simulink model "soccer_strategy"  (R2018a)
settings: Solver=FixedStepDiscrete  StartTime=0.0  StopTime=inf  FixedStep=0.01  RelTol=1e-3
InitFcn:
  | soccer_strategy_setup
model workspace (MAT data in the model file):
  SL_ROS_VariableLengthArrays_MaxSizes.CommonInfo.ArrayTruncateAction = 'EmitWarning'
  SL_ROS_VariableLengthArrays_MaxSizes.MsgTypeMap = containers.Map
  SL_ROS_VariableLengthArrays_MaxSizes.MsgTypeMap.serialization.keys = {'sensor_msgs/Image'}
  SL_ROS_VariableLengthArrays_MaxSizes.MsgTypeMap.serialization.values{1}(1).PropertyName = 'Data'
  SL_ROS_VariableLengthArrays_MaxSizes.MsgTypeMap.serialization.values{1}(1).DataType = 'uint8'
  SL_ROS_VariableLengthArrays_MaxSizes.MsgTypeMap.serialization.values{1}(1).MaxLength = 921600
  SL_ROS_VariableLengthArrays_MaxSizes.MsgTypeMap.serialization.values{1}(2).PropertyName = 'Encoding'
  SL_ROS_VariableLengthArrays_MaxSizes.MsgTypeMap.serialization.values{1}(2).DataType = 'uint8'
  SL_ROS_VariableLengthArrays_MaxSizes.MsgTypeMap.serialization.values{1}(2).MaxLength = 128
  SL_ROS_VariableLengthArrays_MaxSizes.MsgTypeMap.serialization.uniformity = 0
  SL_ROS_VariableLengthArrays_MaxSizes.MsgTypeMap.serialization.keyType = 'char'
  SL_ROS_VariableLengthArrays_MaxSizes.MsgTypeMap.serialization.valueType = 'any'
  ctrlParam1 = 1
  ctrlParam2 = 1.5
  sampleTime = 0.01
values from neighbouring files (symbols this model uses):
  feetGain = 0.1    [soccer_strategy_setup.m]
  forearmGain = 1.5    [soccer_strategy_setup.m]
  hipCalveGain = 1    [soccer_strategy_setup.m]
  kneeGain = 2    [soccer_strategy_setup.m]
  motorCalibration = [      0;      0;      0.05;     0.05;      0;      0;      0;      0;      0;      0;      0;      0;      0;      0;      0;      0;      0;      0;      0;      0]    [soccer_strategy_calibration.m]    (also in soccer_strategy_setup.m = [0;0;0;0;0;0;0;0;0;0;0;0;0;0;0;0;0;0;0;0])
undefined symbols (not defined in the file or in its folder): DiscIntNeverNeededParam, manual, ready, ready_armsback, standing
libraries: robotlib x8, dspsrcs4 x7, simulink x4, simulink_extras x3, robotcorelib x1
settings Model: Creator=scastro  LastModifiedBy=daniel
settings OptimizationCC: PassReuseOutputArgsAs=Individual arguments  EfficientMapNaN2IntZero=off  MaxStackSize=64
settings DebuggingCC: ParameterTunabilityLossMsg=error
settings HardwareCC: ProdBitPerPointer=32  ProdBitPerSizeT=32  ProdBitPerPtrDiffT=32  ProdLargestAtomicFloat=None  ProdIntDivRoundTo=Undefined  ProdEndianess=Unspecified  ProdWordSize=32  ProdHWDeviceType=Generic->Unspecified (assume 32-bit Generic)  TargetBitPerLong=64  TargetBitPerPointer=64  TargetBitPerSizeT=64  TargetBitPerPtrDiffT=64  TargetLongLongMode=on  TargetIntDivRoundTo=Zero  TargetEndianess=LittleEndian  TargetWordSize=64  TargetHWDeviceType=MATLAB Host  ProdEqTarget=off
settings RTWCC: SystemTargetFile=ert.tlc  HardwareBoard=Robot Operating System (ROS)  TLCOptions="-aInlineSetEventsForThisBaseRateFcn=TLC_FALSE -aSuppressMultiTaskScheduler=TLC_FALSE  -aRateBasedStepFcn=0"  TemplateMakefile=ert_default_tmf  GenerateReport=on  Toolchain=Catkin  IncludeHyperlinkInReport=on  LaunchReport=on  TargetLang=C++  GenerateTraceInfo=on  GenerateTraceReport=on  GenerateTraceReportSl=on  GenerateTraceReportSf=on  GenerateTraceReportEml=on
settings CodeAppCC: ForceParamTrailComments=on  IgnoreCustomStorageClasses=off  MaxIdLength=128  OperatorAnnotations=on  SimulinkDataObjDesc=on  SFDataObjDesc=on  InsertBlockDesc=on
settings ERTTargetCC: MultiInstanceERTCode=on  CodeInterfacePackaging=C++ class  SupportVariableSizeSignals=on  RootIOFormat=Structure reference

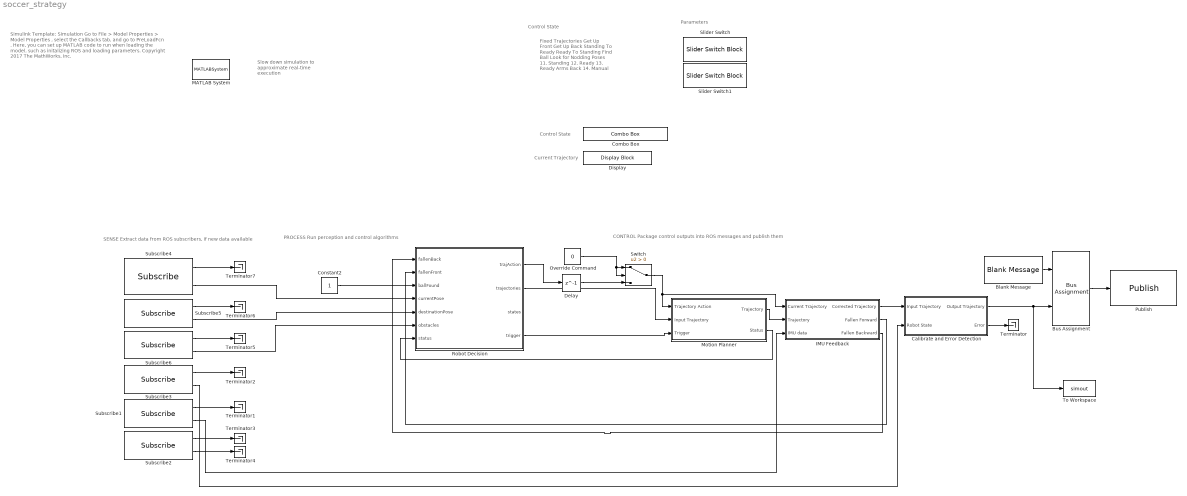
== system soccer_strategy ==
  note: Control State
  note: Control State
  note: Fixed Trajectories
      | Get Up Front
      | Get Up Back
      | Standing To Ready
      | Ready To Standing
      | Find Ball
      | Look for Nodding
      | Poses
      | 11. Standing
      | 12. Ready
      | 13. Ready Arms Back
      | 14. Manual
  note: Simulink Template: Simulation
      |
      | Go to File > Model Properties > Model Properties , select the Callbacks tab, and go to PreLoadFcn .
      |
      | Here, you can set up MATLAB code to run when loading the model, such as initalizing ROS and loading parameters.
      |
      | Copyright 2017 The MathWorks, Inc.
  note: Slow down simulation to approximate real-time execution
  note: PROCESS
      | Run perception and control algorithms
  note: SENSE
      | Extract data from ROS subscribers, if new data available
  note: CONTROL
      | Package control outputs into ROS messages and publish them
  note: Current Trajectory
  note: Parameters
  Blank Message : robotlib/Blank Message  SourceLibraryInfo=This block requires Robotics System Toolbox  messageType=soccer_msgs/RobotGoal  SampleTime=inf
      settings: SourceProductBaseCode=RO
  Bus Assignment : BusAssignment  AssignedSignals=Trajectories
  Calibrate and Error Detection : Subsystem
  Combo Box : ComboBox  WebBlockId=1770  LabelPosition=Hide  SelectedLabel=Autonomous
      settings: Values={{'Get Up Front', 'Get Up Back', 'Standing To Ready', 'Ready To Standing', 'Find Ball', 'Autonomous', 'Standing Pose', 'Ready Pose', 'Look For Nodding', 'Manual', 'Custom Trajectory'}, [1 2 3 4 5 0 11 12 6 13 9]}
  Constant2 : Constant
  Delay : Delay  DelayLength=1
  Display : DisplayBlock  WebBlockId=1772  LabelPosition=Hide
  IMU Feedback : Subsystem
  MATLAB System : MATLABSystem  System=ExampleHelperSimulationRateControl  SampleTime=sampleTime
      mask Type: ExampleHelperSimulationRateControl
      mask Display: disp('Rate Control');
  Motion Planner : Subsystem
  Override Command : Constant  Value=0
  Publish : robotlib/Publish  SourceLibraryInfo=This block requires Robotics System Toolbox  topicSource=Select from ROS network  topic=/robotGoal  messageType=soccer_msgs/RobotGoal  messageQueueLength=1
      settings: SourceProductBaseCode=RO
  Robot Decision : Stateflow chart  TreatAsAtomicUnit=on
  Slider Switch : SliderSwitchBlock  WebBlockId=2006
      settings: Values={{'Off', 'On'}, [0 1]}
  Slider Switch1 : SliderSwitchBlock  WebBlockId=2012
      settings: Values={{'Off', 'On'}, [0 1]}
  Subscribe1 : robotlib/Subscribe  SourceLibraryInfo=This block requires Robotics System Toolbox  topicSource=Select from ROS network  topic=/soccerbot/imu  messageType=sensor_msgs/Imu  sampleTime=-1  messageQueueLength=1
      settings: SourceProductBaseCode=RO
  Subscribe2 : robotlib/Subscribe  SourceLibraryInfo=This block requires Robotics System Toolbox  topicSource=Select from ROS network  topic=/game_state  messageType=team_communication/game_state  sampleTime=-1  messageQueueLength=1
      settings: SourceProductBaseCode=RO
  Subscribe3 : robotlib/Subscribe  SourceLibraryInfo=This block requires Robotics System Toolbox  topicSource=Select from ROS network  topic=/soccerbot/robotState  messageType=soccer_msgs/RobotState  sampleTime=-1  messageQueueLength=1
      settings: SourceProductBaseCode=RO
  Subscribe4 : robotlib/Subscribe  SourceLibraryInfo=This block requires Robotics System Toolbox  topicSource=Specify your own  topic=/soccerbot/currentPose  messageType=geometry_msgs/Pose2D  sampleTime=-1  messageQueueLength=1
      settings: SourceProductBaseCode=RO
  Subscribe5 : robotlib/Subscribe  SourceLibraryInfo=This block requires Robotics System Toolbox  topicSource=Specify your own  topic=/soccerbot/destinationPose  messageType=geometry_msgs/Pose2D  sampleTime=-1  messageQueueLength=1
      settings: SourceProductBaseCode=RO
  Subscribe6 : robotlib/Subscribe  SourceLibraryInfo=This block requires Robotics System Toolbox  topicSource=Specify your own  topic=/soccer_field/obstacles  messageType=soccer_msgs/RobotObstacleArray  sampleTime=-1  messageQueueLength=1
      settings: SourceProductBaseCode=RO
  Switch : Switch  Criteria=u2 > Threshold
  Terminator{,1..7} (8 alike) : Terminator
  To Workspace : ToWorkspace  VariableName=simout  SaveFormat=Timeseries  SampleTime=-1
  wires:
  Calibrate and Error Detection/1(Output Trajectory) -> To Workspace/1, Bus Assignment/2
  Bus Assignment/1 -> Publish/1
  Blank Message/1 -> Bus Assignment/1
  Constant2/1 -> Robot Decision/3(ballFound)
  Robot Decision/4(trigger) -> Motion Planner/3(Trigger)
  Motion Planner/1(Trajectory) -> IMU Feedback/2(Trajectory)
  IMU Feedback/1(Corrected Trajectory) -> Calibrate and Error Detection/1(Input Trajectory)
  Subscribe1/1 -> Terminator1/1
  IMU Feedback/2(Fallen Forward) -> Robot Decision/2(fallenFront)
  IMU Feedback/3(Fallen Backward) -> Robot Decision/1(fallenBack)
  Robot Decision/1(trajAction) -> Delay/1
  Override Command/1 -> Switch/2, Switch/1
  Switch/1 -> IMU Feedback/1(Current Trajectory), Motion Planner/1(Trajectory Action)
  Robot Decision/2(trajectories) -> Motion Planner/2(Input Trajectory)
  Delay/1 -> Switch/3
  Subscribe1/2 -> IMU Feedback/3(IMU data)
  Subscribe2/2 -> Terminator4/1
  Subscribe2/1 -> Terminator3/1
  Motion Planner/2(Status) -> Robot Decision/7(status)
  Subscribe4/2 -> Robot Decision/4(currentPose)
  Subscribe5/2 -> Robot Decision/5(destinationPose)
  Subscribe3/1 -> Terminator2/1
  Subscribe3/2 -> Calibrate and Error Detection/2(Robot State)
  Calibrate and Error Detection/2(Error) -> Terminator/1
  Subscribe6/2 -> Robot Decision/6(obstacles)
  Subscribe6/1 -> Terminator5/1
  Subscribe5/1 -> Terminator6/1
  Subscribe4/1 -> Terminator7/1

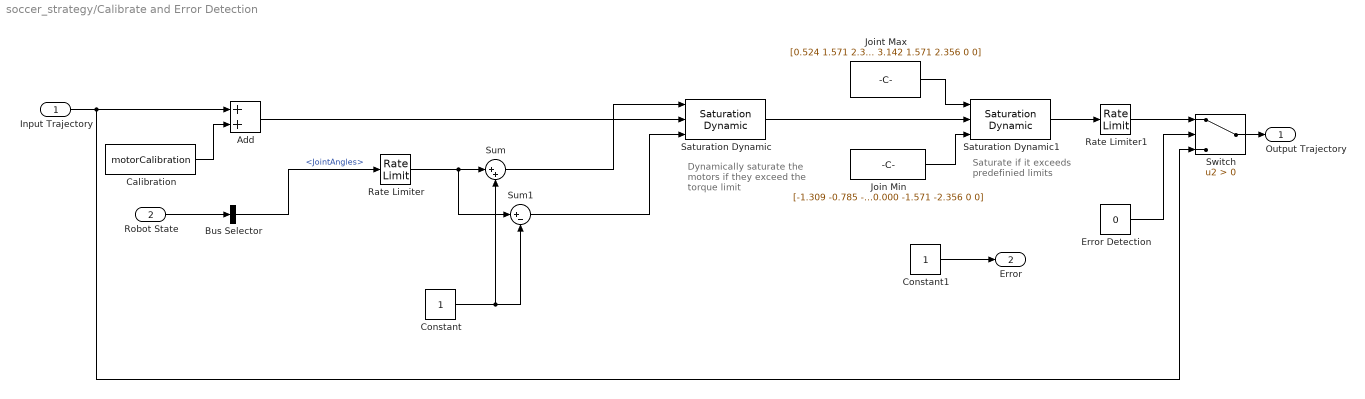
== system soccer_strategy/Calibrate and Error Detection ==
  note: Dynamically saturate the motors if they exceed the torque limit
  note: Saturate if it exceeds predefinied limits
  Input Trajectory : Inport
  Robot State : Inport  Port=2
  Add : Sum
  Bus Selector : BusSelector  OutputSignals=JointAngles
  Calibration : Constant  Value=motorCalibration  OutDataTypeStr=single
  Constant : Constant
  Constant1 : Constant
  Error Detection : Constant  Value=0
  Join Min : Constant  Value=|
      | [-1.309
      | -0.785
      | -0.785
      | -2.793
      | -0.785
      | -0.785
      | -1.309
      | -0.785
      | -0.785
      | -2.793
      | -0.785
      | -0.785
      | -1.571
      | 0.000
      | -1.571
      | 0.000
      | -1.571
      | -2.356
      | 0
      | 0]
  Joint Max : Constant  Value=|
      | [0.524
      | 1.571
      | 2.356
      | 0.000
      | 1.571
      | 0.785
      | 0.524
      | 1.571
      | 2.356
      | 0.000
      | 1.571
      | 0.785
      | 3.927
      | 3.142
      | 3.927
      | 3.142
      | 1.571
      | 2.356
      | 0
      | 0]
  Rate Limiter : RateLimiter  SampleTimeMode=inherited
  Rate Limiter1 : RateLimiter  RisingSlewLimit=15  FallingSlewLimit=-20  SampleTimeMode=inherited
  Saturation Dynamic : simulink/Discontinuities/Saturation Dynamic  OutMin=[]  OutMax=[]  OutDataTypeStr=Inherit: Same as second input  OutDataType=fixdt(1, 16)  OutScaling=2^-10  DoSatur=off
  Saturation Dynamic1 : simulink/Discontinuities/Saturation Dynamic  OutMin=[]  OutMax=[]  OutDataTypeStr=Inherit: Same as second input  OutDataType=fixdt(1, 16)  OutScaling=2^-10  DoSatur=off
  Sum : Sum  Inputs=|++
  Sum1 : Sum  Inputs=|+-
  Switch : Switch  Criteria=u2 > Threshold
  Output Trajectory : Outport
  Error : Outport  Port=2
  wires:
  Calibration/1 -> Add/2
  Saturation Dynamic/1 -> Saturation Dynamic1/2
  Robot State/1 -> Bus Selector/1
  Bus Selector/1 -> Rate Limiter/1  "<JointAngles>"
  Add/1 -> Saturation Dynamic/2
  Rate Limiter/1 -> Sum1/1, Sum/1
  Sum/1 -> Saturation Dynamic/1
  Constant/1 -> Sum1/2, Sum/2
  Sum1/1 -> Saturation Dynamic/3
  Saturation Dynamic1/1 -> Rate Limiter1/1
  Join Min/1 -> Saturation Dynamic1/3
  Joint Max/1 -> Saturation Dynamic1/1
  Constant1/1 -> Error/1
  Error Detection/1 -> Switch/2
  Rate Limiter1/1 -> Switch/1
  Switch/1 -> Output Trajectory/1
  Input Trajectory/1 -> Add/1, Switch/3

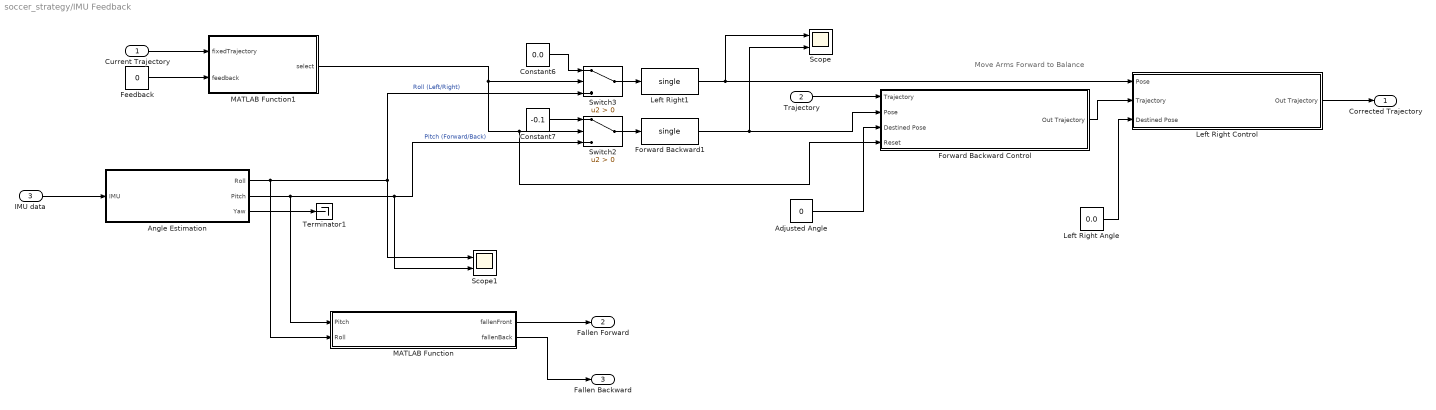
== system soccer_strategy/IMU Feedback ==
  note: Move Arms Forward to Balance
  Current Trajectory : Inport  SampleTime=0.01
  Trajectory : Inport  Port=2  OutDataTypeStr=single
  IMU data : Inport  Port=3
  Adjusted Angle : Constant  Value=0  OutDataTypeStr=single
  Angle Estimation : Subsystem  Variant=on  VariantControl=Variant1  OverrideUsingVariant=Variant
  Constant6 : Constant  Value=0.0
  Constant7 : Constant  Value=-0.1
  Feedback : Constant  Value=0
  Forward Backward Control : Subsystem
  Forward Backward1 : DataTypeConversion  OutDataTypeStr=single
  Left Right Angle : Constant  Value=0.0  OutDataTypeStr=single
  Left Right Control : Subsystem
  Left Right1 : DataTypeConversion  OutDataTypeStr=single
  MATLAB Function : MATLAB Function  TreatAsAtomicUnit=on
  MATLAB Function1 : MATLAB Function  TreatAsAtomicUnit=on
  Scope : Scope  NumInputPorts=2
  Scope1 : Scope  NumInputPorts=2
  Switch2 : Switch  Criteria=u2 > Threshold
  Switch3 : Switch  Criteria=u2 > Threshold
  Terminator1 : Terminator
  Corrected Trajectory : Outport
  Fallen Forward : Outport  Port=2
  Fallen Backward : Outport  Port=3
  wires:
  Trajectory/1 -> Forward Backward Control/1(Trajectory)
  Adjusted Angle/1 -> Forward Backward Control/3(Destined Pose)
  Left Right Angle/1 -> Left Right Control/3(Destined Pose)
  Left Right Control/1(Out Trajectory) -> Corrected Trajectory/1
  Switch2/1 -> Forward Backward1/1
  Switch3/1 -> Left Right1/1
  Constant6/1 -> Switch3/1
  Constant7/1 -> Switch2/1
  Left Right1/1 -> Scope/1, Left Right Control/1(Pose)
  Current Trajectory/1 -> MATLAB Function1/1(fixedTrajectory)
  Angle Estimation/3(" Yaw") -> Terminator1/1
  MATLAB Function/1(fallenFront) -> Fallen Forward/1
  MATLAB Function/2(fallenBack) -> Fallen Backward/1
  Angle Estimation/1(" Roll") -> MATLAB Function/2(Roll), Switch3/3, Scope1/1  "Roll (Left/Right)"
  IMU data/1 -> Angle Estimation/1("IMU ")
  Forward Backward1/1 -> Scope/2, Forward Backward Control/2(Pose)
  Angle Estimation/2(" Pitch") -> Switch2/3, Scope1/2, MATLAB Function/1(Pitch)  "Pitch (Forward/Back)"
  MATLAB Function1/1(select) -> Forward Backward Control/4(Reset), Switch2/2, Switch3/2
  Forward Backward Control/1(Out Trajectory) -> Left Right Control/2(Trajectory)
  Feedback/1 -> MATLAB Function1/2(feedback)

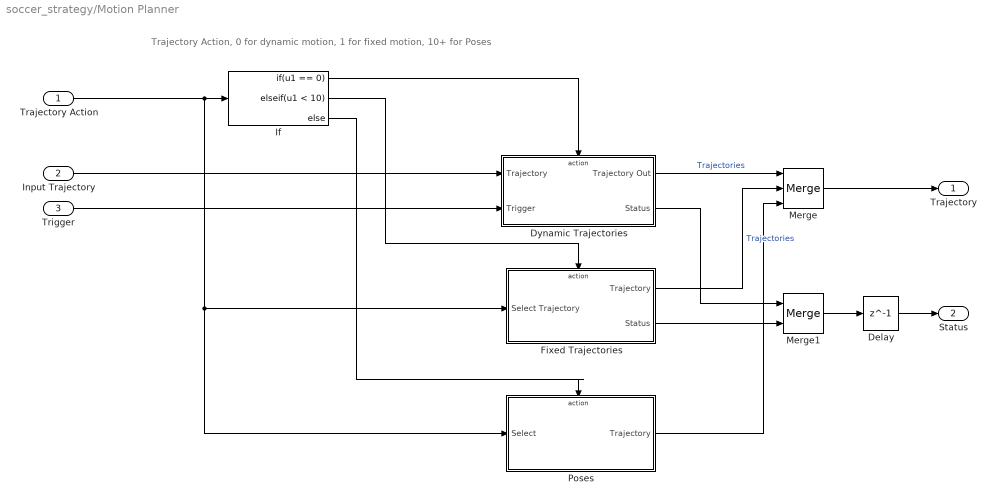
== system soccer_strategy/Motion Planner ==
  note: Trajectory Action, 0 for dynamic motion, 1 for fixed motion, 10+ for Poses
  Trajectory Action : Inport  SampleTime=0.01
  Input Trajectory : Inport  Port=2  PortDimensions=[10000 20]
  Trigger : Inport  Port=3
  Delay : Delay  DelayLength=1
  Dynamic Trajectories : Subsystem  TreatAsAtomicUnit=on
  Fixed Trajectories : Subsystem  TreatAsAtomicUnit=on
  If : If  IfExpression=u1 == 0  ElseIfExpressions=u1 < 10
  Merge : Merge  Inputs=3
  Merge1 : Merge
  Poses : Subsystem  TreatAsAtomicUnit=on
  Trajectory : Outport
  Status : Outport  Port=2
  wires:
  Dynamic Trajectories/1(Trajectory Out) -> Merge/1  "Trajectories"
  If/1 -> Dynamic Trajectories/Action
  Fixed Trajectories/1(Trajectory) -> Merge/2  "Trajectories"
  If/2 -> Fixed Trajectories/Action
  Input Trajectory/1 -> Dynamic Trajectories/1(Trajectory)
  Merge/1 -> Trajectory/1
  Fixed Trajectories/2(Status) -> Merge1/2
  Dynamic Trajectories/2(Status) -> Merge1/1
  Trajectory Action/1 -> Poses/1(Select), Fixed Trajectories/1(Select Trajectory), If/1
  Merge1/1 -> Delay/1
  Poses/1(Trajectory) -> Merge/3
  If/3 -> Poses/Action
  Trigger/1 -> Dynamic Trajectories/2(Trigger)
  Delay/1 -> Status/1

== system soccer_strategy/Robot Decision/StatusOk.calculateTrajectory ==
  currentPose : Inport  OutDataTypeStr=Bus: SL_Bus_soccer_strategy_geometry_msgs_Pose2D  PortDimensions=1
  destinationPose : Inport  Port=2  OutDataTypeStr=Bus: SL_Bus_soccer_strategy_geometry_msgs_Pose2D  PortDimensions=1
  obstacles : Inport  Port=3  OutDataTypeStr=Bus: SL_Bus_soccer_strategy_soccer_msgs_RobotObstacleArray  PortDimensions=1
  f : TriggerPort  TriggerType=function-call  VariantControl=(inherit)
      settings: CopyFcn=Stateflow.SLINSF.SimulinkMan.removeBlockPreDeleteFcn  PreDeleteFcn=Stateflow.SLINSF.SimulinkMan.unsafePredeleteFcn
  MATLAB System : MATLABSystem  System=findtrajectorysystem  outputduration=100  SimulateUsing=Interpreted execution
      mask Type: findtrajectorysystem
      mask Display:
      | disp('findtrajectorysystem');
      | port_label('input',1,'currentPose');
      | port_label('input',2,'destinationPose');
      | port_label('input',3,'obstacles');
      | port_label('output',1,'trajectory');
      | port_label('output',2,'states');
  trajectories : Outport
  states : Outport  Port=2
  wires:
  currentPose/1 -> MATLAB System/1
  destinationPose/1 -> MATLAB System/2
  obstacles/1 -> MATLAB System/3
  MATLAB System/1 -> trajectories/1
  MATLAB System/2 -> states/1

== system soccer_strategy/IMU Feedback/Angle Estimation ==
  "IMU " : Inport
  Complementary FIlter : Subsystem  VariantControl=Variant1
  Direct Information : Subsystem  VariantControl=Variant
  " Roll" : Outport
  " Pitch" : Outport  Port=2
  " Yaw" : Outport  Port=3

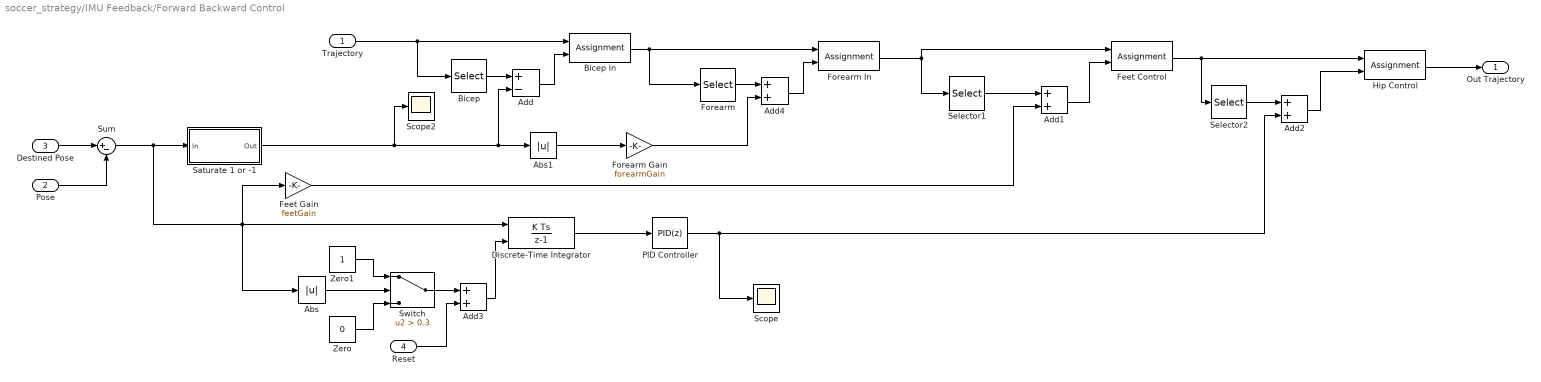
== system soccer_strategy/IMU Feedback/Forward Backward Control ==
  Trajectory : Inport
  Pose : Inport  Port=2
  Destined Pose : Inport  Port=3  OutDataTypeStr=single
  Reset : Inport  Port=4
  Abs : Abs
  Abs1 : Abs
  Add : Sum  Inputs=+-
  Add{1..4} (4 alike) : Sum
  Bicep : Selector  InputPortWidth=20  IndexOptions=Index vector (dialog)  Indices=[13 15]  OutputSizes=1
  Bicep In : Assignment  DiagnosticForDimensions=Warning  IndexOptions=Index vector (dialog)  Indices=[13 15]  OutputSizes=1
  Discrete-Time Integrator : DiscreteIntegrator  gainval=1  ExternalReset=level  SampleTime=-1  LimitOutput=on  UpperSaturationLimit=0.2  LowerSaturationLimit=-0.2  ICPrevOutput=DiscIntNeverNeededParam  ICPrevScaledInput=DiscIntNeverNeededParam
  Feet Control : Assignment  DiagnosticForDimensions=Warning  IndexOptions=Index vector (dialog)  Indices=[5 11]  OutputSizes=1
  "Feet Gain " : Gain  Gain=feetGain
  Forearm : Selector  InputPortWidth=20  IndexOptions=Index vector (dialog)  Indices=[14 16]  OutputSizes=1
  Forearm Gain : Gain  Gain=forearmGain
  Forearm In : Assignment  DiagnosticForDimensions=Warning  IndexOptions=Index vector (dialog)  Indices=[14 16]  OutputSizes=1
  Hip Control : Assignment  DiagnosticForDimensions=Warning  IndexOptions=Index vector (dialog)  Indices=[3 9]  OutputSizes=1
  PID Controller : simulink/Continuous/PID Controller  Controller=PID  TimeDomain=Discrete-time  SampleTime=-1  IntegratorMethod=Forward Euler  FilterMethod=Forward Euler  Form=Parallel  UseFilter=on  ControllerParametersSource=internal  P=2  I=5  D=0  N=100  InitialConditionSource=internal  InitialConditionForIntegrator=0  InitialConditionForFilter=0  ExternalReset=none  LimitOutput=off  UpperSaturationLimit=inf  LowerSaturationLimit=-inf  LinearizeAsGain=on  AntiWindupMode=none  Kb=1  TrackingMode=off  Kt=1  PParamMin=[]  PParamMax=[]  IParamMin=[]  IParamMax=[]  DParamMin=[]  DParamMax=[]  NParamMin=[]  NParamMax=[]  KbParamMin=[]  KbParamMax=[]  KtParamMin=[]  KtParamMax=[]  POutMin=[]  POutMax=[]  IOutMin=[]  IOutMax=[]  DOutMin=[]  DOutMax=[]  NOutMin=[]  NOutMax=[]  KbOutMin=[]  KbOutMax=[]  KtOutMin=[]  KtOutMax=[]  IntegratorOutMin=[]  IntegratorOutMax=[]  FilterOutMin=[]  FilterOutMax=[]  SumOutMin=[]  SumOutMax=[]  SumI1OutMin=[]  SumI1OutMax=[]  SumI2OutMin=[]  SumI2OutMax=[]  SumI3OutMin=[]  SumI3OutMax=[]  SumDOutMin=[]  SumDOutMax=[]  SaturationOutMin=[]  SaturationOutMax=[]  IntegratorContinuousStateAttributes=''  IntegratorStateMustResolveToSignalObject=off  IntegratorRTWStateStorageClass=Auto  FilterContinuousStateAttributes=''  FilterStateMustResolveToSignalObject=off  FilterRTWStateStorageClass=Auto  DifferentiatorICPrevScaledInput=0  DifferentiatorOutMin=[]  DifferentiatorOutMax=[]  FilterDiffOutCoefMin=[]  FilterDiffOutCoefMax=[]  SumDenOutMin=[]  SumDenOutMax=[]  SumNumOutMin=[]  SumNumOutMax=[]  ReciprocalOutMin=[]  ReciprocalOutMax=[]  DivideOutMin=[]  DivideOutMax=[]  TunerSelectOption=Transfer Function Based (PID Tuner App)
  Saturate 1 or -1 : Subsystem
  Scope : Scope
  Scope2 : Scope
  Selector1 : Selector  InputPortWidth=20  IndexOptions=Index vector (dialog)  Indices=[5 11]  OutputSizes=1
  Selector2 : Selector  InputPortWidth=20  IndexOptions=Index vector (dialog)  Indices=[3 9]  OutputSizes=1
  Sum : Sum  Inputs=|+-
  Switch : Switch  Criteria=u2 > Threshold  Threshold=0.3
  Zero : Constant  Value=0
  Zero1 : Constant
  Out Trajectory : Outport
  wires:
  Trajectory/1 -> Bicep/1, Bicep In/1
  "Feet Gain "/1 -> Add1/2
  Forearm In/1 -> Selector1/1, Feet Control/1
  Add/1 -> Bicep In/2
  Bicep/1 -> Add/1
  Add1/1 -> Feet Control/2
  Destined Pose/1 -> Sum/1
  Selector1/1 -> Add1/1
  Feet Control/1 -> Selector2/1, Hip Control/1
  Add2/1 -> Hip Control/2
  Selector2/1 -> Add2/1
  Hip Control/1 -> Out Trajectory/1
  Saturate 1 or -1/1(Out) -> Abs1/1, Add/2, Scope2/1
  Pose/1 -> Sum/2
  Abs/1 -> Switch/2
  Zero/1 -> Switch/3
  Zero1/1 -> Switch/1
  Reset/1 -> Add3/2
  Switch/1 -> Add3/1
  Add3/1 -> Discrete-Time Integrator/2
  Forearm/1 -> Add4/1
  Add4/1 -> Forearm In/2
  Abs1/1 -> Forearm Gain/1
  Bicep In/1 -> Forearm/1, Forearm In/1
  Forearm Gain/1 -> Add4/2
  Discrete-Time Integrator/1 -> PID Controller/1
  Sum/1 -> Discrete-Time Integrator/1, Abs/1, "Feet Gain "/1, Saturate 1 or -1/1(In)
  PID Controller/1 -> Scope/1, Add2/2

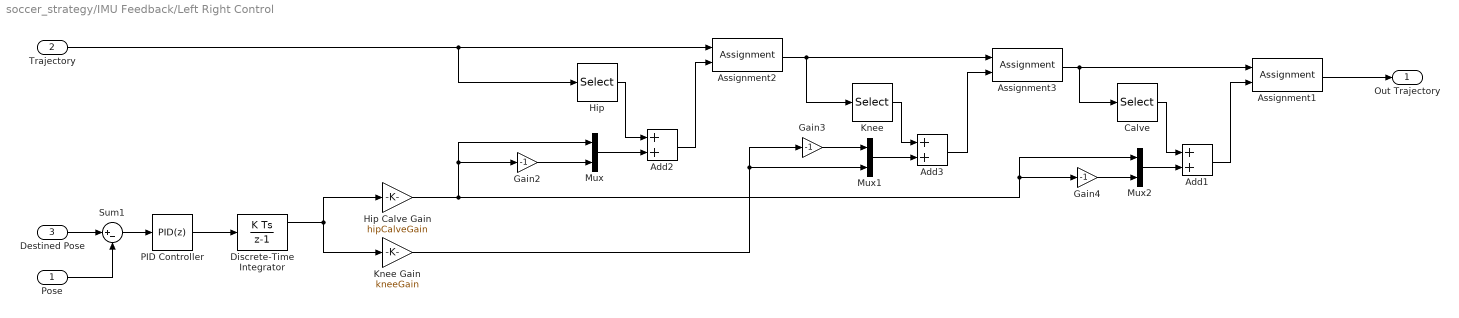
== system soccer_strategy/IMU Feedback/Left Right Control ==
  Pose : Inport
  Trajectory : Inport  Port=2
  Destined Pose : Inport  Port=3
  Add1 : Sum
  Add2 : Sum
  Add3 : Sum
  Assignment1 : Assignment  DiagnosticForDimensions=Warning  IndexOptions=Index vector (dialog)  Indices=[5,11]  OutputSizes=1
  Assignment2 : Assignment  DiagnosticForDimensions=Warning  IndexOptions=Index vector (dialog)  Indices=[3,9]  OutputSizes=1
  Assignment3 : Assignment  DiagnosticForDimensions=Warning  IndexOptions=Index vector (dialog)  Indices=[4,10]  OutputSizes=1
  Calve : Selector  InputPortWidth=20  IndexOptions=Index vector (dialog)  Indices=[5,11]  OutputSizes=1
  Discrete-Time Integrator : DiscreteIntegrator  gainval=1  SampleTime=-1  LimitOutput=on  UpperSaturationLimit=0.08  LowerSaturationLimit=-0.08  ShowSaturationPort=on  ICPrevOutput=DiscIntNeverNeededParam  ICPrevScaledInput=DiscIntNeverNeededParam
  Gain2 : Gain  Gain=-1
  Gain3 : Gain  Gain=-1
  Gain4 : Gain  Gain=-1
  Hip : Selector  InputPortWidth=20  IndexOptions=Index vector (dialog)  Indices=[3,9]  OutputSizes=1
  Hip Calve Gain : Gain  Gain=hipCalveGain
  Knee : Selector  InputPortWidth=20  IndexOptions=Index vector (dialog)  Indices=[4,10]  OutputSizes=1
  Knee Gain : Gain  Gain=kneeGain
  Mux : Mux  Inputs=2
  Mux1 : Mux  Inputs=2
  Mux2 : Mux  Inputs=2
  PID Controller : simulink/Continuous/PID Controller  Controller=PID  TimeDomain=Discrete-time  SampleTime=-1  IntegratorMethod=Forward Euler  FilterMethod=Forward Euler  Form=Parallel  UseFilter=on  ControllerParametersSource=internal  P=1  I=1  D=0  N=100  InitialConditionSource=internal  InitialConditionForIntegrator=0  InitialConditionForFilter=0  ExternalReset=none  LimitOutput=off  UpperSaturationLimit=inf  LowerSaturationLimit=-inf  LinearizeAsGain=on  AntiWindupMode=none  Kb=1  TrackingMode=off  Kt=1  PParamMin=[]  PParamMax=[]  IParamMin=[]  IParamMax=[]  DParamMin=[]  DParamMax=[]  NParamMin=[]  NParamMax=[]  KbParamMin=[]  KbParamMax=[]  KtParamMin=[]  KtParamMax=[]  POutMin=[]  POutMax=[]  IOutMin=[]  IOutMax=[]  DOutMin=[]  DOutMax=[]  NOutMin=[]  NOutMax=[]  KbOutMin=[]  KbOutMax=[]  KtOutMin=[]  KtOutMax=[]  IntegratorOutMin=[]  IntegratorOutMax=[]  FilterOutMin=[]  FilterOutMax=[]  SumOutMin=[]  SumOutMax=[]  SumI1OutMin=[]  SumI1OutMax=[]  SumI2OutMin=[]  SumI2OutMax=[]  SumI3OutMin=[]  SumI3OutMax=[]  SumDOutMin=[]  SumDOutMax=[]  SaturationOutMin=[]  SaturationOutMax=[]  IntegratorContinuousStateAttributes=''  IntegratorStateMustResolveToSignalObject=off  IntegratorRTWStateStorageClass=Auto  FilterContinuousStateAttributes=''  FilterStateMustResolveToSignalObject=off  FilterRTWStateStorageClass=Auto  DifferentiatorICPrevScaledInput=0  DifferentiatorOutMin=[]  DifferentiatorOutMax=[]  FilterDiffOutCoefMin=[]  FilterDiffOutCoefMax=[]  SumDenOutMin=[]  SumDenOutMax=[]  SumNumOutMin=[]  SumNumOutMax=[]  ReciprocalOutMin=[]  ReciprocalOutMax=[]  DivideOutMin=[]  DivideOutMax=[]  TunerSelectOption=Transfer Function Based (PID Tuner App)
  Sum1 : Sum  Inputs=|+-
  Out Trajectory : Outport
  wires:
  Pose/1 -> Sum1/2
  Destined Pose/1 -> Sum1/1
  Assignment2/1 -> Knee/1, Assignment3/1
  Add2/1 -> Assignment2/2
  Sum1/1 -> PID Controller/1
  Knee/1 -> Add3/1
  Hip/1 -> Add2/1
  Add3/1 -> Assignment3/2
  Trajectory/1 -> Hip/1, Assignment2/1
  Assignment3/1 -> Calve/1, Assignment1/1
  Assignment1/1 -> Out Trajectory/1
  Calve/1 -> Add1/1
  Add1/1 -> Assignment1/2
  Mux/1 -> Add2/2
  Mux1/1 -> Add3/2
  Knee Gain/1 -> Mux1/2, Gain3/1
  Mux2/1 -> Add1/2
  Discrete-Time Integrator/1 -> Hip Calve Gain/1, Knee Gain/1
  Gain3/1 -> Mux1/1
  Hip Calve Gain/1 -> Mux2/1, Gain4/1, Gain2/1, Mux/1
  PID Controller/1 -> Discrete-Time Integrator/1
  Gain2/1 -> Mux/2
  Gain4/1 -> Mux2/2

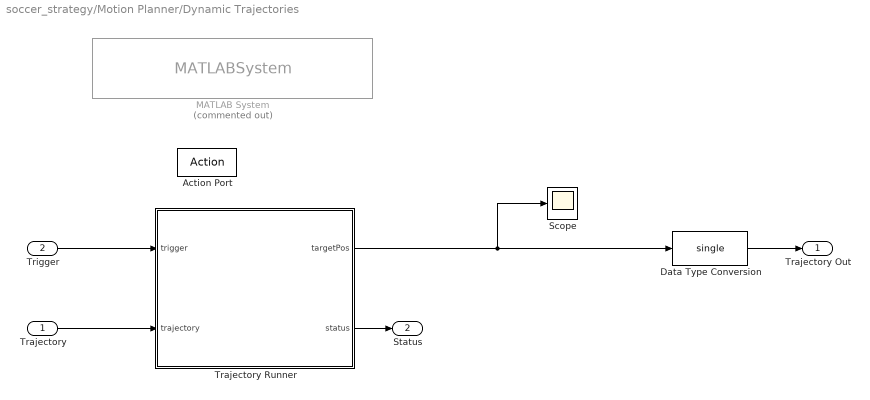
== system soccer_strategy/Motion Planner/Dynamic Trajectories ==
  Trajectory : Inport
  Trigger : Inport  Port=2
  Action Port : ActionPort  ActionType=then
  Data Type Conversion : DataTypeConversion  OutDataTypeStr=single
  MATLAB System : MATLABSystem  Commented=on  System=BipedalRobotSystemObject  statusUpdateTimeBeforeEnd=5  SimulateUsing=Interpreted execution
      mask Type: BipedalRobotSystemObject
      mask Display:
      | disp('BipedalRobotSystemObject');
      | port_label('input',1,'waypoints');
      | port_label('input',2,'trigger');
      | port_label('output',1,'trajectories');
      | port_label('output',2,'status');
  Scope : Scope
  Trajectory Runner : Stateflow chart  TreatAsAtomicUnit=on
  Trajectory Out : Outport  PortDimensions=[1,20]
  Status : Outport  Port=2
  wires:
  Trajectory/1 -> Trajectory Runner/2(trajectory)
  Data Type Conversion/1 -> Trajectory Out/1
  Trajectory Runner/1(targetPos) -> Scope/1, Data Type Conversion/1
  Trajectory Runner/2(status) -> Status/1
  Trigger/1 -> Trajectory Runner/1(trigger)

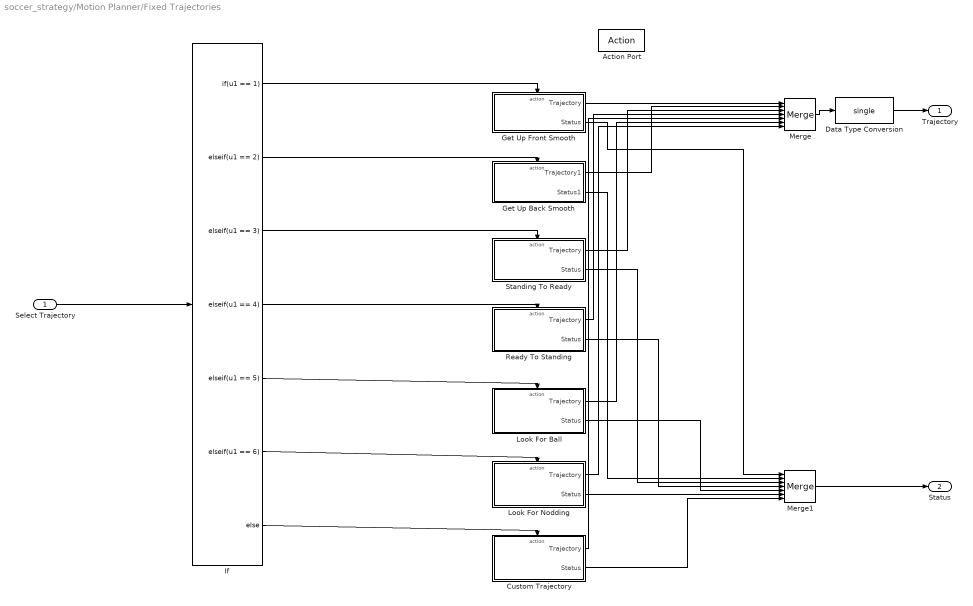
== system soccer_strategy/Motion Planner/Fixed Trajectories ==
  Select Trajectory : Inport  SampleTime=0.01
  Action Port : ActionPort  InitializeStates=reset  ActionType=elseif
  Custom Trajectory : Subsystem  TreatAsAtomicUnit=on
  Data Type Conversion : DataTypeConversion  OutDataTypeStr=single
  Get Up Back Smooth : Subsystem  TreatAsAtomicUnit=on
  Get Up Front Smooth : Subsystem  TreatAsAtomicUnit=on
  If : If  IfExpression=u1 == 1  ElseIfExpressions=u1 == 2, u1 == 3, u1 == 4, u1 == 5, u1 == 6
  Look For Ball : Subsystem  TreatAsAtomicUnit=on
  Look For Nodding : Subsystem  TreatAsAtomicUnit=on
  Merge : Merge  Inputs=7
  Merge1 : Merge  Inputs=7
  Ready To Standing : Subsystem  TreatAsAtomicUnit=on
  Standing To Ready : Subsystem  TreatAsAtomicUnit=on
  Trajectory : Outport
  Status : Outport  Port=2
  wires:
  Data Type Conversion/1 -> Trajectory/1
  Merge/1 -> Data Type Conversion/1
  If/2 -> Get Up Back Smooth/Action
  Merge1/1 -> Status/1
  Select Trajectory/1 -> If/1
  If/1 -> Get Up Front Smooth/Action
  Get Up Front Smooth/1(Trajectory) -> Merge/1
  Get Up Front Smooth/2(Status) -> Merge1/1
  Get Up Back Smooth/1(Trajectory1) -> Merge/2
  Get Up Back Smooth/2(Status1) -> Merge1/2
  If/3 -> Standing To Ready/Action
  If/4 -> Ready To Standing/Action
  If/7 -> Custom Trajectory/Action
  Standing To Ready/1(Trajectory) -> Merge/3
  Ready To Standing/1(Trajectory) -> Merge/4
  Custom Trajectory/1(Trajectory) -> Merge/5
  Standing To Ready/2(Status) -> Merge1/3
  Ready To Standing/2(Status) -> Merge1/4
  Custom Trajectory/2(Status) -> Merge1/7
  If/5 -> Look For Ball/Action
  Look For Ball/1(Trajectory) -> Merge/6
  Look For Ball/2(Status) -> Merge1/5
  If/6 -> Look For Nodding/Action
  Look For Nodding/1(Trajectory) -> Merge/7
  Look For Nodding/2(Status) -> Merge1/6

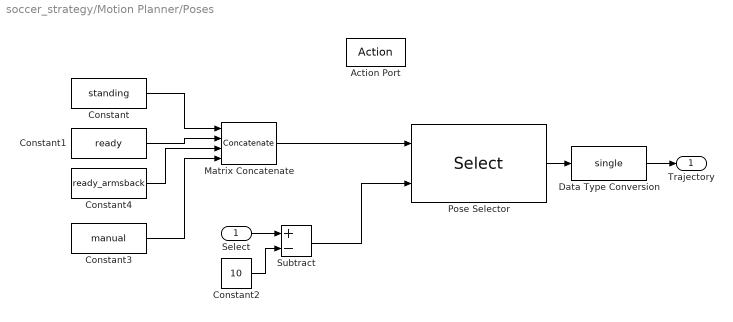
== system soccer_strategy/Motion Planner/Poses ==
  Select : Inport
  Action Port : ActionPort  InitializeStates=reset  ActionType=else
  Constant : Constant  Value=standing  VectorParams1D=off
  Constant1 : Constant  Value=ready  VectorParams1D=off
  Constant2 : Constant  Value=10
  Constant3 : Constant  Value=manual  VectorParams1D=off
  Constant4 : Constant  Value=ready_armsback  VectorParams1D=off
  Data Type Conversion : DataTypeConversion  OutDataTypeStr=single
  Matrix Concatenate : Concatenate  NumInputs=4  Mode=Multidimensional array
  Pose Selector : Selector  NumberOfDimensions=2  InputPortWidth=3  IndexOptions=Index vector (port),Select all  Indices=[1 3],1  OutputSizes=1,1
  Subtract : Sum  Inputs=+-
  Trajectory : Outport
  wires:
  Constant1/1 -> Matrix Concatenate/2
  Matrix Concatenate/1 -> Pose Selector/1
  Constant/1 -> Matrix Concatenate/1
  Subtract/1 -> Pose Selector/2
  Select/1 -> Subtract/1
  Constant2/1 -> Subtract/2
  Pose Selector/1 -> Data Type Conversion/1
  Data Type Conversion/1 -> Trajectory/1
  Constant3/1 -> Matrix Concatenate/4
  Constant4/1 -> Matrix Concatenate/3

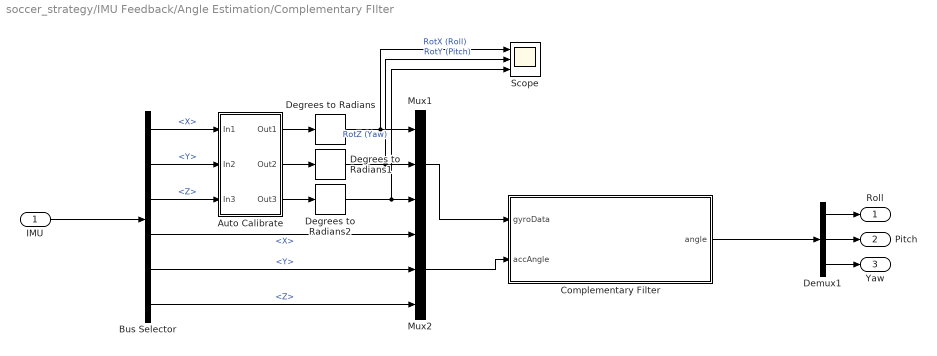
== system soccer_strategy/IMU Feedback/Angle Estimation/Complementary FIlter ==
  "IMU " : Inport
  Auto Calibrate : Subsystem
  Bus Selector : BusSelector  OutputSignals=AngularVelocity.X,AngularVelocity.Y,AngularVelocity.Z,LinearAcceleration.X,LinearAcceleration.Y,LinearAcceleration.Z
  Complementary Filter : MATLAB Function  TreatAsAtomicUnit=on
      settings: MinAlgLoopOccurrences=on
  Degrees to Radians : simulink_extras/Transformations/Degrees to Radians
  Degrees to Radians1 : simulink_extras/Transformations/Degrees to Radians
  Degrees to Radians2 : simulink_extras/Transformations/Degrees to Radians
  Demux1 : Demux  Outputs=3
  Mux1 : Mux  Inputs=3
  Mux2 : Mux  Inputs=3
  Scope : Scope  NumInputPorts=3
  " Roll" : Outport
  " Pitch" : Outport  Port=2
  " Yaw" : Outport  Port=3
  wires:
  "IMU "/1 -> Bus Selector/1
  Bus Selector/1 -> Auto Calibrate/1(In1)  "<X>"
  Bus Selector/4 -> Mux2/1  "<X>"
  Bus Selector/5 -> Mux2/2  "<Y>"
  Bus Selector/6 -> Mux2/3  "<Z>"
  Complementary Filter/1(angle) -> Demux1/1
  Mux1/1 -> Complementary Filter/1(gyroData)
  Mux2/1 -> Complementary Filter/2(accAngle)
  Demux1/1 -> " Roll"/1
  Demux1/2 -> " Pitch"/1
  Demux1/3 -> " Yaw"/1
  Bus Selector/2 -> Auto Calibrate/2(In2)  "<Y>"
  Bus Selector/3 -> Auto Calibrate/3(In3)  "<Z>"
  Auto Calibrate/1(Out1) -> Degrees to Radians/1
  Auto Calibrate/2(Out2) -> Degrees to Radians1/1
  Auto Calibrate/3(Out3) -> Degrees to Radians2/1
  Degrees to Radians/1 -> Scope/1, Mux1/1  "RotX (Roll)"
  Degrees to Radians1/1 -> Mux1/2, Scope/2  "RotY (Pitch)"
  Degrees to Radians2/1 -> Mux1/3, Scope/3  "RotZ (Yaw)"

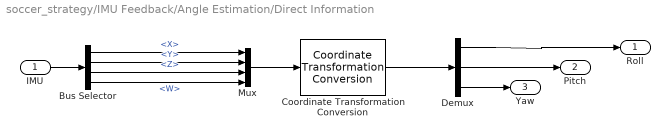
== system soccer_strategy/IMU Feedback/Angle Estimation/Direct Information ==
  "IMU " : Inport
  Bus Selector : BusSelector  OutputSignals=Orientation.X,Orientation.Y,Orientation.Z,Orientation.W
  Coordinate Transformation Conversion : robotcorelib/Coordinate Transformation Conversion  InputRepresentation=Quaternion  InputEulerSequence=ZYX  ShowTrVecInputPort=on  OutputRepresentation=Euler Angles  OutputEulerSequence=XYZ  ShowTrVecOutputPort=on  SimulateUsing=Interpreted execution
      settings: SourceProductBaseCode=RO
  Demux : Demux  Outputs=3
  Mux : Mux
  " Roll" : Outport
  " Pitch" : Outport  Port=2
  " Yaw" : Outport  Port=3
  wires:
  "IMU "/1 -> Bus Selector/1
  Bus Selector/2 -> Mux/2  "<Y>"
  Bus Selector/4 -> Mux/4  "<W>"
  Coordinate Transformation Conversion/1 -> Demux/1
  Mux/1 -> Coordinate Transformation Conversion/1
  Bus Selector/3 -> Mux/3  "<Z>"
  Bus Selector/1 -> Mux/1  "<X>"
  Demux/2 -> " Pitch"/1
  Demux/3 -> " Yaw"/1
  Demux/1 -> " Roll"/1

== system soccer_strategy/IMU Feedback/Forward Backward Control/Saturate 1 or -1 ==
  In : Inport
  Gain : Gain  Gain=-1
  Switch1 : Switch  Criteria=u2 > Threshold  Threshold=0.25
  Switch2 : Switch  Criteria=u2 > Threshold  Threshold=0.25
  Zero : Constant  Value=0  OutDataTypeStr=single
  Zero1 : Constant  OutDataTypeStr=single
  Zero2 : Constant  Value=-1  OutDataTypeStr=single
  Out : Outport
  wires:
  In/1 -> Switch1/2, Gain/1
  Switch1/1 -> Switch2/3
  Gain/1 -> Switch2/2
  Zero/1 -> Switch1/3
  Zero1/1 -> Switch1/1
  Zero2/1 -> Switch2/1
  Switch2/1 -> Out/1

== system soccer_strategy/Motion Planner/Fixed Trajectories/Custom Trajectory ==
  Action Port : ActionPort  InitializeStates=reset  ActionType=else
  Signal : dspsrcs4/Signal From Workspace  X=customTrajectory.Data  Ts=0.01  nsamps=1  OutputAfterFinalValue=Cyclic repetition  ignoreOrWarnInputAndFrameLengths=off  OutputFrames=off
  Step : Step  Time=customTrajectory.time(end)  SampleTime=0.01
  Trajectory : Outport
  Status : Outport  Port=2
  wires:
  Signal/1 -> Trajectory/1
  Step/1 -> Status/1

== system soccer_strategy/Motion Planner/Fixed Trajectories/Get Up Back Smooth ==
  Action Port : ActionPort  InitializeStates=reset  ActionType=elseif
  Signal1 : dspsrcs4/Signal From Workspace  X=getupbacksmooth.Data  Ts=0.01  nsamps=1  OutputAfterFinalValue=Cyclic repetition  ignoreOrWarnInputAndFrameLengths=off  OutputFrames=off
  Step1 : Step  Time=getupbacksmooth.time(end)  SampleTime=0.01
  Trajectory1 : Outport
  Status1 : Outport  Port=2
  wires:
  Step1/1 -> Status1/1
  Signal1/1 -> Trajectory1/1

== system soccer_strategy/Motion Planner/Fixed Trajectories/Get Up Front Smooth ==
  Action Port : ActionPort  InitializeStates=reset  ActionType=then
  Signal : dspsrcs4/Signal From Workspace  X=getupfrontsmooth.Data  Ts=0.01  nsamps=1  OutputAfterFinalValue=Cyclic repetition  ignoreOrWarnInputAndFrameLengths=off  OutputFrames=off
  Step : Step  Time=getupfrontsmooth.time(end)  SampleTime=0.01
  Trajectory : Outport
  Status : Outport  Port=2
  wires:
  Signal/1 -> Trajectory/1
  Step/1 -> Status/1

== system soccer_strategy/Motion Planner/Fixed Trajectories/Look For Ball ==
  Action Port : ActionPort  InitializeStates=reset  ActionType=elseif
  Signal : dspsrcs4/Signal From Workspace  X=headShakingTrajectory.Data  Ts=0.01  nsamps=1  OutputAfterFinalValue=Cyclic repetition  ignoreOrWarnInputAndFrameLengths=off  OutputFrames=off
  Step : Step  Time=headShakingTrajectory.time(end)  SampleTime=0.01
  Trajectory : Outport
  Status : Outport  Port=2
  wires:
  Signal/1 -> Trajectory/1
  Step/1 -> Status/1

== system soccer_strategy/Motion Planner/Fixed Trajectories/Look For Nodding ==
  Action Port : ActionPort  InitializeStates=reset  ActionType=elseif
  Signal : dspsrcs4/Signal From Workspace  X=headNoddingTrajectory.Data  Ts=0.01  nsamps=1  OutputAfterFinalValue=Cyclic repetition  ignoreOrWarnInputAndFrameLengths=off  OutputFrames=off
  Step : Step  Time=headNoddingTrajectory.time(end)  SampleTime=0.01
  Trajectory : Outport
  Status : Outport  Port=2
  wires:
  Signal/1 -> Trajectory/1
  Step/1 -> Status/1

== system soccer_strategy/Motion Planner/Fixed Trajectories/Ready To Standing ==
  Action Port : ActionPort  InitializeStates=reset  ActionType=elseif
  Signal : dspsrcs4/Signal From Workspace  X=readytostanding.Data  Ts=0.01  nsamps=1  OutputAfterFinalValue=Holding final value  ignoreOrWarnInputAndFrameLengths=off  OutputFrames=off
  Step : Step  Time=readytostanding.time(end)  SampleTime=0.01
  Trajectory : Outport
  Status : Outport  Port=2
  wires:
  Step/1 -> Status/1
  Signal/1 -> Trajectory/1

== system soccer_strategy/Motion Planner/Fixed Trajectories/Standing To Ready ==
  Action Port : ActionPort  InitializeStates=reset  ActionType=elseif
  Signal : dspsrcs4/Signal From Workspace  X=standingtoready.Data  Ts=0.01  nsamps=1  OutputAfterFinalValue=Holding final value  ignoreOrWarnInputAndFrameLengths=off  OutputFrames=off
  Step : Step  Time=standingtoready.time(end)  SampleTime=0.01
  Trajectory : Outport
  Status : Outport  Port=2
  wires:
  Signal/1 -> Trajectory/1
  Step/1 -> Status/1

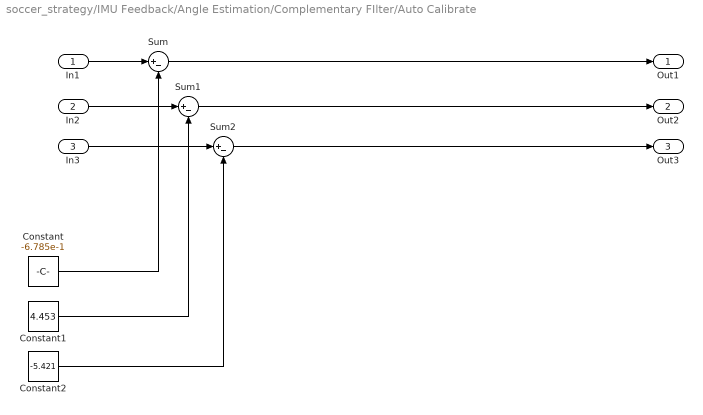
== system soccer_strategy/IMU Feedback/Angle Estimation/Complementary FIlter/Auto Calibrate ==
  In1 : Inport
  In2 : Inport  Port=2
  In3 : Inport  Port=3
  Constant : Constant  Value=-6.785e-1
  Constant1 : Constant  Value=4.453
  Constant2 : Constant  Value=-5.421
  Sum : Sum  Inputs=|+-
  Sum1 : Sum  Inputs=|+-
  Sum2 : Sum  Inputs=|+-
  Out1 : Outport
  Out2 : Outport  Port=2
  Out3 : Outport  Port=3
  wires:
  Sum2/1 -> Out3/1
  Sum1/1 -> Out2/1
  Sum/1 -> Out1/1
  In1/1 -> Sum/1
  In2/1 -> Sum1/1
  In3/1 -> Sum2/1
  Constant/1 -> Sum/2
  Constant1/1 -> Sum1/2
  Constant2/1 -> Sum2/2

== matlab function soccer_strategy/IMU Feedback/MATLAB Function1 ==
  data: fixedTrajectory input; select output; feedback input
function select = selectBalanceAlgorithm(fixedTrajectory, feedback)
    if (~feedback)
        select = 1;
        return;
    end

    if (fixedTrajectory ~= 11 && fixedTrajectory ~= 12 && fixedTrajectory ~= 5 && fixedTrajectory ~= 6)
        select = 1;
    else
        select = 0;
    end
end

== matlab function soccer_strategy/IMU Feedback/MATLAB Function ==
  data: Pitch input; fallenFront output; fallenBack output; Roll input
function [fallenFront, fallenBack] = determineFallenDirection(Pitch, Roll)
    fallenFront = 0;
    fallenBack = 0;

    if(Pitch < -0.5)
        fallenBack = 1;
    elseif (Pitch > 0.5)
        fallenFront = 1;
    end
end

== stateflow chart soccer_strategy/Robot Decision ==
  state StatusOk
    state Ready
      entry: trajAction = 13;
      trajectories = zeros(10000,20);
      states = zeros(10000,1);
    state LookForBall
      entry: trajAction = 5; trigger = 0;
    state PrepareToWalk
      entry: trajAction = 5;
    state Walking
      entry: trajAction = 0;
      [trajectories,states] = calculateTrajectory(currentPose, destinationPose, obstacles);
      trigger = 1;
    state [trajectories,states] = calculateTrajectory(currentPose,destinationPose,obstacles) [function]
    (default) -> Ready
    Ready -> LookForBall : [after(3,sec)]
    Walking -> LookForBall : [status == 1 && after(1,sec)]
    LookForBall -> LookForBall [order 1] : [ballFound==0 && after(10,sec)]
    LookForBall -> PrepareToWalk [order 2] : [ballFound == 1 && after(1,sec)]
    PrepareToWalk -> Walking : [status == 1 && after(1,sec)]
  state FallenFront
    entry: trajAction = 1;
  state FallenBack
    entry: trajAction = 2;
  FallenFront -> StatusOk [order 1] : [status == 1 && fallenBack ~= 1 && fallenFront ~= 1]
  (default) -> StatusOk
  FallenFront -> FallenFront [order 3] : [status == 1 && fallenFront == 1]
  StatusOk -> FallenFront [order 2] : [fallenFront == 1 && after(3, sec)]
  FallenFront -> FallenBack [order 2] : [status == 1 && fallenBack == 1]
  FallenBack -> FallenFront [order 2] : [status == 1 && fallenFront == 1]
  StatusOk -> FallenBack [order 1] : [fallenBack == 1 && after(3, sec)]
  FallenBack -> FallenBack [order 1] : [status == 1 && fallenBack== 1]
  data: currentPose function_input Bus: SL_Bus_soccer_strategy_geometry_msgs_Pose2D size=1; destinationPose function_input Bus: SL_Bus_soccer_strategy_geometry_msgs_Pose2D size=1; obstacles function_input Bus: SL_Bus_soccer_strategy_soccer_msgs_RobotObstacleArray size=1; trajectories function_output; states function_output; fallenBack input; fallenFront input; ballFound input; currentPose input; destinationPose input; obstacles input; status input; trajAction output; trajectories output; states output; trigger output; trajectoryTemp local

== matlab function soccer_strategy/IMU Feedback/Angle Estimation/Complementary FIlter/Complementary Filter ==
  data: angle output; gyroData input; accAngle input
function angle = ComplementaryFilter( gyroData, accAngle)
    dt = 0.01;
    
    persistent temp_angle;
    if isempty(temp_angle)
        temp_angle = zeros(3,1);
    end
    
    gyroRatio = 0;
    
    Rx = accAngle(1);
    Ry = accAngle(2);
    Rz = accAngle(3);
    angle = temp_angle;
%     angle(1) = 1 * atan2(Ry, -Rz); % Roll
%     angle(2) = 1 * atan2(Rx, -Rz); % Pitch

    angle(1) = gyroRatio * (angle(2) + gyroData(2) * dt) + (1 - gyroRatio) * -atan2(Ry, -Rz); % Roll
    angle(2) = gyroRatio * (angle(3) + gyroData(3) * dt) + (1 - gyroRatio) * -atan2(Rx, -Rz); % Pitch

== stateflow chart soccer_strategy/Motion Planner/Dynamic Trajectories/Trajectory Runner ==
  state StepOnTrajectory
    entry:
    currentState=currentState+1;
  state SetConfiguration
    entry,during:
    targetPos=trajectory(currentState,:);
    status=0;
  state EndTrajectory
    entry:
    currentState=1;
    status=1;
  StepOnTrajectory -> SetConfiguration
  SetConfiguration -> StepOnTrajectory [order 1] : [after(0.01,sec)]
  EndTrajectory -> SetConfiguration : [trigger==1]
  SetConfiguration -> EndTrajectory [order 2] : [currentState == length(trajectory)-1]
  (default) -> EndTrajectory
  data: targetPos output; status output; trigger input; trajectory input; currentState local
